simulink model "lab_2_3"  (R2023b)
settings: Solver=FixedStepAuto  StartTime=0.0  StopTime=10.0  FixedStep=solver_time  RelTol=1e-3
undefined symbols (not defined in the file): A, C, x_0
settings Model: Creator=nsukh  LastModifiedBy=nsukh

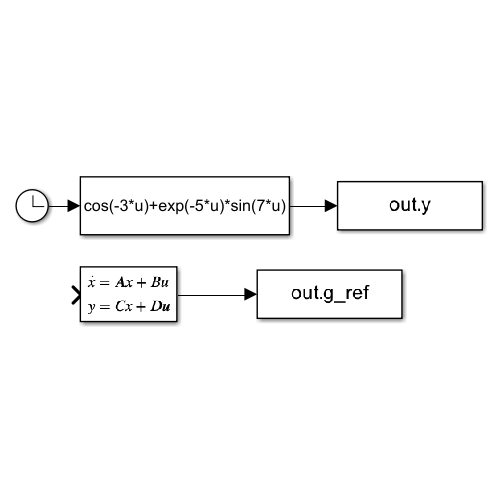
[thumbnail: Simulink's stored preview of the top-level diagram]
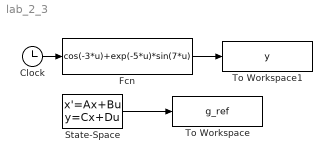
== system lab_2_3 ==
  Clock : Clock
  Fcn : Fcn  Expr=cos(-3*u)+exp(-5*u)*sin(7*u)
  State-Space : StateSpace  A=A  B=[0,0,0,0;0,0,0,0;0,0,0,0;0,0,0,0]  C=C  D=[0,0,0,0]  InitialCondition=x_0
  To Workspace : ToWorkspace  VariableName=g_ref  SaveFormat=Timeseries  SampleTime=-1
  To Workspace1 : ToWorkspace  VariableName=y  SaveFormat=Timeseries  SampleTime=-1
  wires:
  Clock/1 -> Fcn/1
  State-Space/1 -> To Workspace/1
  Fcn/1 -> To Workspace1/1
